simulink model "multiroom_heating_system"  (R2023b)
settings: Solver=VariableStepAuto  StartTime=0.0  StopTime=10  RelTol=1e-3
model workspace (MAT data in the model file):
  A = [0  0.3  0.4  0.3; 0.3  0  0.5  0; 0.4  0.5  0  0.3; 0.3  0  0.3  0]
  b = [0.3; 0.2; 0.5; 0.4]
  c = [9; 7; 11; 7]
  diff = [1; 1; 1; 1]
  get = [17; 17; 17; 17]
  max_temp = 20
  min_temp = 15
  off = [20; 20; 20; 20]
  on = [19; 19; 19; 19]
  u = 6
  x_0 = [16.5; 16.5; 16.5; 16.5]
settings Model: Creator=williamstar
settings ModelReferenceCC: EnableRefExpFcnMdlSchedulingChecks=on

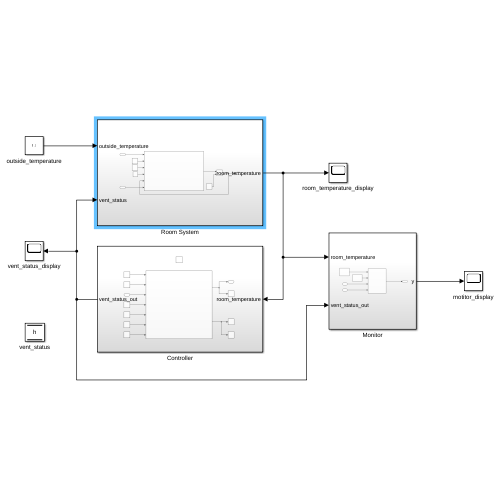
[thumbnail: Simulink's stored preview of the top-level diagram]
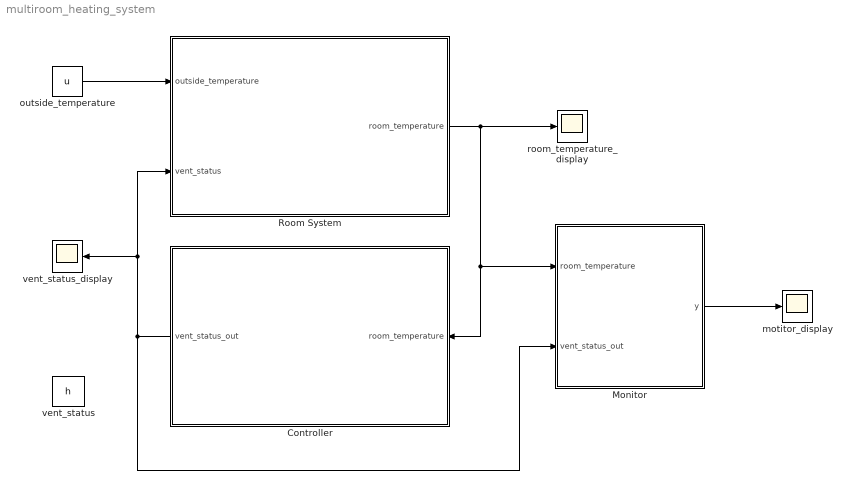
== system multiroom_heating_system ==
  Controller : Subsystem
  Monitor : Subsystem
  Room System : Subsystem
  motitor_display : Scope
  outside_temperature : Constant  Value=u
  room_temperature_display : Scope
  vent_status : DataStoreMemory  DataStoreName=h  WriteAfterWriteMsg=warning  InitialValue=[0;0;0;0]  ShowAdditionalParam=off
  vent_status_display : Scope
  wires:
  outside_temperature/1 -> Room System/1(outside_temperature)
  Room System/1(room_temperature) -> Controller/1(room_temperature), Monitor/1(room_temperature), room_temperature_display/1
  Controller/1(vent_status_out) -> Room System/2(vent_status), vent_status_display/1, Monitor/2(vent_status_out)
  Monitor/1(y) -> motitor_display/1

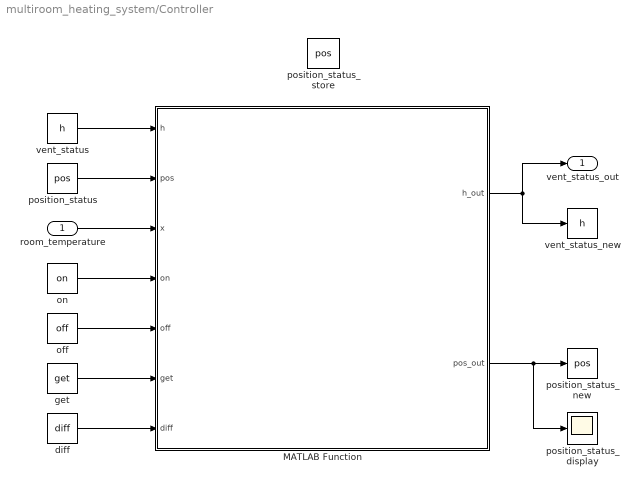
== system multiroom_heating_system/Controller ==
  room_temperature : Inport
  MATLAB Function : MATLAB Function  TreatAsAtomicUnit=on
  diff : Constant  Value=diff
  get : Constant  Value=get
  off : Constant  Value=off
  on : Constant  Value=on
  position_status : DataStoreRead  DataStoreName=pos  IndexOptions=Index vector (dialog)  Indices=1  OutputSizes=1
  position_status_display : Scope
  position_status_new : DataStoreWrite  DataStoreName=pos  IndexOptions=Index vector (dialog)  Indices=1  OutputSizes=1
  position_status_store : DataStoreMemory  DataStoreName=pos  WriteAfterWriteMsg=warning  InitialValue=[0;1;1;0]  ShowAdditionalParam=off
  vent_status : DataStoreRead  DataStoreName=h  IndexOptions=Index vector (dialog)  Indices=1  OutputSizes=1
  vent_status_new : DataStoreWrite  DataStoreName=h  IndexOptions=Index vector (dialog)  Indices=1  OutputSizes=1
  vent_status_out : Outport
  wires:
  room_temperature/1 -> MATLAB Function/3(x)
  on/1 -> MATLAB Function/4(on)
  off/1 -> MATLAB Function/5(off)
  get/1 -> MATLAB Function/6(get)
  diff/1 -> MATLAB Function/7(diff)
  vent_status/1 -> MATLAB Function/1(h)
  position_status/1 -> MATLAB Function/2(pos)
  MATLAB Function/2(pos_out) -> position_status_new/1, position_status_display/1
  MATLAB Function/1(h_out) -> vent_status_new/1, vent_status_out/1

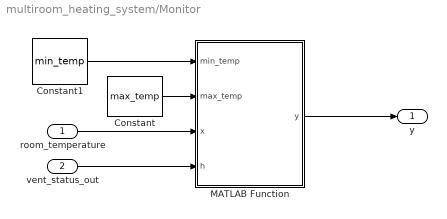
== system multiroom_heating_system/Monitor ==
  room_temperature : Inport
  vent_status_out : Inport  Port=2
  Constant : Constant  Value=max_temp
  Constant1 : Constant  Value=min_temp
  MATLAB Function : MATLAB Function  TreatAsAtomicUnit=on
  y : Outport
  wires:
  room_temperature/1 -> MATLAB Function/3(x)
  vent_status_out/1 -> MATLAB Function/4(h)
  MATLAB Function/1(y) -> y/1
  Constant1/1 -> MATLAB Function/1(min_temp)
  Constant/1 -> MATLAB Function/2(max_temp)

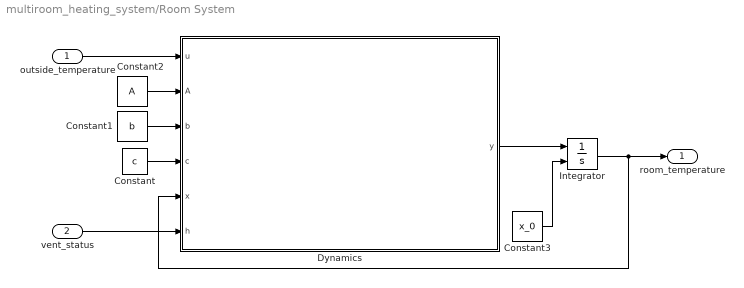
== system multiroom_heating_system/Room System ==
  outside_temperature : Inport
  vent_status : Inport  Port=2
  Constant : Constant  Value=c
  Constant1 : Constant  Value=b
  Constant2 : Constant  Value=A
  Constant3 : Constant  Value=x_0
  Dynamics : MATLAB Function  TreatAsAtomicUnit=on
  Integrator : Integrator  InitialConditionSource=external
  room_temperature : Outport
  wires:
  outside_temperature/1 -> Dynamics/1(u)
  Constant/1 -> Dynamics/4(c)
  Constant1/1 -> Dynamics/3(b)
  Constant2/1 -> Dynamics/2(A)
  vent_status/1 -> Dynamics/6(h)
  Dynamics/1(y) -> Integrator/1
  Constant3/1 -> Integrator/2
  Integrator/1 -> Dynamics/5(x), room_temperature/1

== matlab function multiroom_heating_system/Controller/MATLAB Function ==
  data: h input; h_out output; pos input; x input; on input; off input; get input; diff input; pos_out output
% function that calculates how vent status should be altered

% h - previous vent status
% pos - previous vent open positions
% x - current room temp
% on - thresholds to open vents
% off - thresholds to close vents
% get - threshold to open a vent in a room & close in another
% diff - threshold of temp diff between room for vent transfer

% h_out - updated vent status
% pos_out - keep track of which room have vents open

function [h_out, pos_out] = fcn(h, pos, x, on, off, get, diff)
    % close / open vents accordingly for each room
    for i = 1:4
        if x(i) >= off(i) && h(i) == 1
            h(i) = 0;
        elseif x(i) <= on(i) && pos(i) == 1
            h(i) = 1;
        end
    end

    % choose to "move" the first vent possible:
    for i = 1:4
        for j = 1:4
            if i ~= j
                 if pos(i) == 0 && pos(j) == 1 && x(i) <= get(i) && x(j) - x(i) >= diff(i)
                    h(i) = 1;
                    h(j) = 0;
                    pos(i) = 1;
                    pos(j) = 0;
                    break
                end
            end
        end
    end

   
    h_out = h;
    pos_out = pos;
end

== matlab function multiroom_heating_system/Room System/Dynamics ==
  data: u input; A input; b input; c input; y output; x input; h input
% Calculate the room dynamics
% according to given formula

% u - outside temp
% A - heat transfer factor between rooms
% b - heat transfer factor from outside
% c - heat transfer factor from heater

% y - current temperate change rate
function y = fcn(u, A, b, c, x, h)
    y = h .* c + (u - x) .* b;
    for i = 1:4
        y(i) = y(i) + A(i,:) * (x - x(i));
    end
end

== matlab function multiroom_heating_system/Monitor/MATLAB Function ==
  data: min_temp input; max_temp input; x input; y output; h input
% function to check if current system state satisfy safety requirements

function y = fcn(min_temp, max_temp, x, h)

    % check if temperature is in bounds 
    % and no more than 2 vents open at the same time
    if any(x < min_temp) || any(x > max_temp) || sum(h==1) > 2
        y = 1;
    else
        y = 0;
    end
    
end
